simulink library "E78TestPack2"  (R2023b)
settings: Solver=VariableStepAuto  StartTime=0.0  StopTime=10.0  RelTol=1e-3
undefined symbols (not defined in the file or in its folder): battery_builder_rtmsupport, gcbh
libraries: E78TestPack2_lib x4
(part 2 of 2)

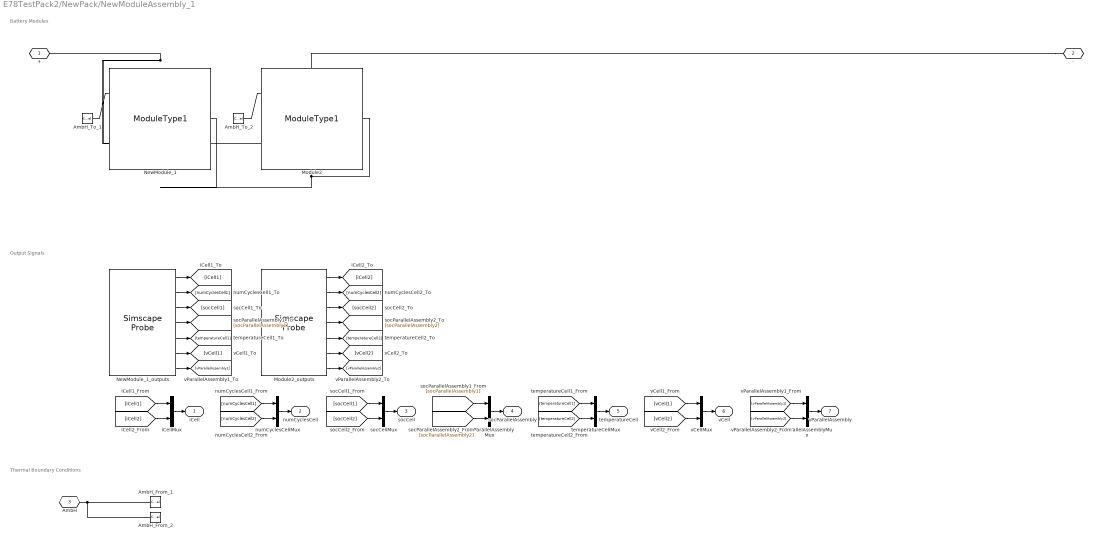
== system E78TestPack2/NewPack/NewModuleAssembly_1 ==
  note: Thermal Boundary Conditions
  note: Output Signals
  note: Battery Modules
  AmbH_From_1 : ConnectionLabel  Label=ambH_1
  AmbH_From_2 : ConnectionLabel  Label=ambH_2
  AmbH_To_1 : ConnectionLabel  Label=ambH_1
  AmbH_To_2 : ConnectionLabel  Label=ambH_2
  Module2 : E78TestPack2_lib/Modules/ModuleType1  SOC_vecCell=[0, .01, .02, .03, .04, .05, .06, .07, .08, .09, .1, .11, .12, .13, .14, .15, .16, .17, .18, .19, .2, .21, .22, .23, .24, .25, .26, .27, .28, .29, .3, .31, .32, .33, .34, .35, .36, .37, .38, .39, .4, .41, .42, .43, .44, .45, .46, .47, .48, .49, .5, .51, .52, .53, .54, .55, .56, .57, .58, .59, .6, .61, .62, .63, .64, .65, .66, .67, .68, .69, .7, .71, .72, .73, .74, .75, .76, .77, .78, .79, .8, .81, .82, .83, .84, .85, .86, .87, .88, .89, .9, .91, .92, .93, .94, .95, .96, .97, .98, .99, 1]  T_vecCell=[-10, 0, 10, 25, 35] degC  V0_matCell=[2.93217, 2.93217, 2.93217, 2.93217, 2.93217; 2.94263, 2.94263, 2.94263, 2.94263, 2.94263; 2.95309, 2.95309, 2.95309, 2.95309, 2.95309; 2.96355, 2.96355, 2.96355, 2.96355, 2.96355; 2.97401, 2.97401, 2.97401, 2.97401, 2.97401; 2.98447, 2.98447, 2.98447, 2.98447, 2.98447; 2.99493, 2.99493, 2.99493, 2.99493, 2.99493; 3.02455, 3.02455, 3.02455, 3.02455, 3.02455; 3.05382, 3.05382, 3.05382, 3.05382, 3.05382; 3.07377, 3.07377, 3.07377, 3.07377, 3.07377; 3.08453, 3.08453, 3.08453, 3.08453, 3.08453; 3.09529, 3.09529, 3.09529, 3.09529, 3.09529; 3.09916, 3.09916, 3.09916, 3.09916, 3.09916; 3.10271, 3.10271, 3.10271, 3.10271, 3.10271; 3.10625, 3.10625, 3.10625, 3.10625, 3.10625; 3.1098, 3.1098, 3.1098, 3.1098, 3.1098; 3.11335, 3.11335, 3.11335, 3.11335, 3.11335; 3.11689, 3.11689, 3.11689, 3.11689, 3.11689; 3.12044, 3.12044, 3.12044, 3.12044, 3.12044; 3.13089, 3.13089, 3.13089, 3.13089, 3.13089; 3.13795, 3.13795, 3.13795, 3.13795, 3.13795; 3.14459, 3.14459, 3.14459, 3.14459, 3.14459; 3.14961, 3.14961, 3.14961, 3.14961, 3.14961; 3.15451, 3.15451, 3.15451, 3.15451, 3.15451; 3.15932, 3.15932, 3.15932, 3.15932, 3.15932; 3.16324, 3.16324, 3.16324, 3.16324, 3.16324; 3.16716, 3.16716, 3.16716, 3.16716, 3.16716; 3.17063, 3.17063, 3.17063, 3.17063, 3.17063; 3.17297, 3.17297, 3.17297, 3.17297, 3.17297; 3.17544, 3.17544, 3.17544, 3.17544, 3.17544; 3.17798, 3.17798, 3.17798, 3.17798, 3.17798; 3.18052, 3.18052, 3.18052, 3.18052, 3.18052; 3.18295, 3.18295, 3.18295, 3.18295, 3.18295; 3.18533, 3.18533, 3.18533, 3.18533, 3.18533; 3.18771, 3.18771, 3.18771, 3.18771, 3.18771; 3.19009, 3.19009, 3.19009, 3.19009, 3.19009; 3.19215, 3.19215, 3.19215, 3.19215, 3.19215; 3.19403, 3.19403, 3.19403, 3.19403, 3.19403; 3.1959, 3.1959, 3.1959, 3.1959, 3.1959; 3.19777, 3.19777, 3.19777, 3.19777, 3.19777; 3.1998, 3.1998, 3.1998, 3.1998, 3.1998; 3.20198, 3.20198, 3.20198, 3.20198, 3.20198; 3.20371, 3.20371, 3.20371, 3.20371, 3.20371; 3.20501, 3.20501, 3.20501, 3.20501, 3.20501; 3.20619, 3.20619, 3.20619, 3.20619, 3.20619; 3.20738, 3.20738, 3.20738, 3.20738, 3.20738; 3.20856, 3.20856, 3.20856, 3.20856, 3.20856; 3.20974, 3.20974, 3.20974, 3.20974, 3.20974; 3.21092, 3.21092, 3.21092, 3.21092, 3.21092; 3.2121, 3.2121, 3.2121, 3.2121, 3.2121; 3.21329, 3.21329, 3.21329, 3.21329, 3.21329; 3.21447, 3.21447, 3.21447, 3.21447, 3.21447; 3.21565, 3.21565, 3.21565, 3.21565, 3.21565; 3.21672, 3.21672, 3.21672, 3.21672, 3.21672; 3.21787, 3.21787, 3.21787, 3.21787, 3.21787; 3.21904, 3.21904, 3.21904, 3.21904, 3.21904; 3.22021, 3.22021, 3.22021, 3.22021, 3.22021; 3.22139, 3.22139, 3.22139, 3.22139, 3.22139; 3.22256, 3.22256, 3.22256, 3.22256, 3.22256; 3.22374, 3.22374, 3.22374, 3.22374, 3.22374; 3.22492, 3.22492, 3.22492, 3.22492, 3.22492; 3.2261, 3.2261, 3.2261, 3.2261, 3.2261; 3.22728, 3.22728, 3.22728, 3.22728, 3.22728; 3.22847, 3.22847, 3.22847, 3.22847, 3.22847; 3.22965, 3.22965, 3.22965, 3.22965, 3.22965; 3.23083, 3.23083, 3.23083, 3.23083, 3.23083; 3.23201, 3.23201, 3.23201, 3.23201, 3.23201; 3.23319, 3.23319, 3.23319, 3.23319, 3.23319; 3.23437, 3.23437, 3.23437, 3.23437, 3.23437; 3.23552, 3.23552, 3.23552, 3.23552, 3.23552; 3.23652, 3.23652, 3.23652, 3.23652, 3.23652; 3.23778, 3.23778, 3.23778, 3.23778, 3.23778; 3.23909, 3.23909, 3.23909, 3.23909, 3.23909; 3.24045, 3.24045, 3.24045, 3.24045, 3.24045; 3.24217, 3.24217, 3.24217, 3.24217, 3.24217; 3.2439, 3.2439, 3.2439, 3.2439, 3.2439; 3.24563, 3.24563, 3.24563, 3.24563, 3.24563; 3.24736, 3.24736, 3.24736, 3.24736, 3.24736; 3.24909, 3.24909, 3.24909, 3.24909, 3.24909; 3.25082, 3.25082, 3.25082, 3.25082, 3.25082; 3.25255, 3.25255, 3.25255, 3.25255, 3.25255; 3.25428, 3.25428, 3.25428, 3.25428, 3.25428; 3.256, 3.256, 3.256, 3.256, 3.256; 3.25774, 3.25774, 3.25774, 3.25774, 3.25774; 3.25951, 3.25951, 3.25951, 3.25951, 3.25951; 3.26116, 3.26116, 3.26116, 3.26116, 3.26116; 3.26238, 3.26238, 3.26238, 3.26238, 3.26238; 3.26307, 3.26307, 3.26307, 3.26307, 3.26307; 3.26352, 3.26352, 3.26352, 3.26352, 3.26352; 3.26396, 3.26396, 3.26396, ...(+502 chars)] V  V_rangeCell=[1.8, Inf] V  R0_matCell=[.07996, .07435, .07218, .00349, .04758; .07879, .07234, .06844, .0033, .01888; .07763, .07033, .0647, .00311, .01407; .07646, .06833, .06096, .00292, .00948; .07529, .06632, .05722, .00272, .0049; .07413, .06432, .05347, .00253, .00119; .07296, .06231, .04973, .00235, .00022; .07278, .06129, .04698, .00233, .00024; .07258, .06024, .0446, .00235, .00024; .0719, .05873, .04247, .00232, .00024; .07075, .05673, .03988, .00223, .00024; .0696, .05474, .03743, .00214, .00024; .06809, .0524, .03472, .00205, .00024; .06657, .05004, .032, .00196, .00024; .06505, .04768, .02927, .00187, .00024; .06353, .04532, .02655, .00181, .00024; .06201, .04298, .02426, .00175, .00024; .06049, .04073, .02215, .00169, .00024; .05897, .03848, .02004, .00164, .00024; .0578, .03658, .01828, .00167, .0006; .05646, .03451, .01635, .00168, .00078; .0551, .03261, .01479, .00168, .00094; .05366, .03068, .01317, .00168, .00101; .0522, .02875, .01154, .00168, .00108; .05075, .02681, .01054, .00167, .00114; .04925, .02502, .01001, .00167, .00116; .04759, .02356, .00948, .00167, .00118; .04591, .02208, .00893, .00167, .00118; .04416, .02054, .00832, .00166, .00112; .04243, .01901, .00772, .00165, .00111; .0407, .01812, .00742, .00164, .00113; .03899, .01727, .0072, .00164, .00115; .03731, .01641, .00697, .00163, .00116; .03563, .01555, .00675, .00163, .00117; .03395, .01474, .00652, .00162, .00119; .03227, .01421, .0063, .00162, .0012; .03067, .01366, .00605, .00161, .00119; .02945, .0131, .00583, .0016, .00118; .02823, .01254, .0058, .00159, .00117; .02701, .01213, .00577, .00159, .00115; .02586, .01192, .00574, .00158, .00115; .02512, .01173, .00573, .00158, .00115; .02436, .01151, .00569, .00158, .00113; .02358, .01127, .00563, .00157, .00109; .02279, .01107, .00557, .00156, .00111; .022, .01096, .0055, .00156, .00112; .02121, .01085, .00544, .00155, .00114; .02046, .01074, .00537, .00154, .00115; .0201, .01063, .00534, .00154, .00117; .01974, .01052, .00531, .00153, .00118; .01938, .01042, .00528, .00153, .00119; .01902, .01031, .00526, .00152, .00121; .01865, .0102, .00523, .00151, .00122; .01829, .01009, .00519, .00151, .00123; .01792, .00998, .00516, .0015, .00124; .01756, .00987, .00513, .0015, .00126; .01735, .00976, .0051, .0015, .00127; .01723, .00967, .00507, .00149, .00128; .01712, .00965, .00504, .00149, .0013; .017, .00963, .00501, .00149, .00131; .01688, .00961, .00498, .00148, .00133; .01676, .00959, .00496, .00148, .00134; .01665, .00957, .00493, .00148, .00135; .01653, .00955, .0049, .00147, .00137; .01641, .00953, .00488, .00147, .00138; .01629, .00951, .00485, .00147, .0014; .01618, .00949, .00482, .00147, .00141; .01606, .00947, .00479, .00146, .00142; .01594, .00945, .00477, .00146, .00143; .01589, .00942, .00474, .00146, .00141; .01586, .00937, .0047, .00145, .00139; .01584, .00934, .00468, .00146, .00139; .01583, .0093, .00466, .00146, .00138; .01581, .00927, .00464, .00147, .00138; .01582, .00926, .00464, .00147, .0014; .01583, .00925, .00464, .00148, .00141; .01583, .00924, .00465, .00149, .00143; .01584, .00923, .00465, .0015, .00145; .01584, .00921, .00465, .0015, .00146; .01585, .00923, .00465, .00151, .00148; .01585, .00925, .00465, .00152, .0015; .01586, .00926, .00465, .00153, .00152; .01587, .00928, .00465, .00153, .00153; .01587, .0093, .00464, .00154, .00155; .01588, .00932, .00463, .00155, .00157; .01589, .00933, .00462, .00155, .00158; .01587, .00933, .00459, .00156, .00157; .01582, .00929, .00453, .00155, .00154; .01576, .00924, .00446, .00154, .00146; .0157, .00919, .00438, .00153, .00132; .01564, .00915, .00431, .00152, .00118; .01558, .0091, .00424, .00151, .00103; .01552, .00905, .00416, .0015, .00089; .01539, .00891, .0041, .00148, .00076; .01518, .00871, .00401, .00144, .00061; .01502, .00857, .00398, .0014, .00051; .01487, .00844, .00396, .00137, .00041; .01501, .0086, .00385, .00136, .00062; .01436, .00795, .00371, .00131, .00087; .01329, .00785, .00411, .00127, .00126; .01299, .00622, .00111, .00104, .00185] Ohm  AHCell=19.487 A*hr  extrapolation_optionCell=simscape.enum.extrapolation.nearest  thermal_massCell=446.4 J/K  AmbientResistance=25 K/W  InterParallelAssemblyThermalResistance=1 K/W  InterParallelAssemblyRadiationArea=1e-3 m^2  InterParallelAssemblyRadiationCoefficient=1e-6 W/(K^4*m^2)  P=1  S=12  NumInterParallelAssemblyThermalConnections=11  InterParallelAssemblyConnectionsMapping=[1, 2, 3, 4, 5, 6, 7, 8, 9, 10, 11; 2, 3, 4, 5, 6, 7, 8, 9, 10, 11, 12]  InterParallelAssemblyCellConnectionsMapping=[1, 1, 1, 1, 1, 1, 1, 1, 1, 1, 1; 1, 1, 1, 1, 1, 1, 1, 1, 1, 1, 1]  iCell_specify=off  iCell_priority=None  iCell=repmat(0, 12, 1) A  iCell_nominal_specify=off  iCell_nominal_unit=A  iCell_nominal_value=1  vCell_specify=off  vCell_priority=None  vCell=repmat(0, 12, 1) V  vCell_nominal_specify=off  vCell_nominal_unit=V  vCell_nominal_value=1  socCell_specify=off  socCell_priority=High  socCell=repmat(1, 12, 1)  socCell_nominal_specify=off  socCell_nominal_unit=1  socCell_nominal_value=1  numCyclesCell_specify=off  numCyclesCell_priority=High  numCyclesCell=repmat(0, 12, 1)  numCyclesCell_nominal_specify=off  numCyclesCell_nominal_unit=1  numCyclesCell_nominal_value=1  temperatureCell_specify=off  temperatureCell_priority=High  temperatureCell=repmat(298.15, 12, 1) K  temperatureCell_nominal_specify=off  temperatureCell_nominal_unit=K  temperatureCell_nominal_value=1  vParallelAssembly_specify=off  vParallelAssembly_priority=None  vParallelAssembly=repmat(0, 12, 1) V  vParallelAssembly_nominal_specify=off  vParallelAssembly_nominal_unit=V  vParallelAssembly_nominal_value=1  socParallelAssembly_specify=off  socParallelAssembly_priority=None  socParallelAssembly=repmat(1, 12, 1)  socParallelAssembly_nominal_specify=off  socParallelAssembly_nominal_unit=1  socParallelAssembly_nominal_value=1
      settings: InternalSimscapePortConfiguration="{\"Bottom\":[{\"id\":\"n\",\"label\":\"-\",\"type\":\"foundation.electrical.electrical\"}],\"Left\":[{\"id\":\"AmbH\",\"label\":\"AmbH\",\"type\":\"foundation.thermal.thermal\"}],\"Right\":[],\"Top\":[{\"id\":\"p\",\"label\":\"+\",\"type\":\"foundation.electrical.electrical\"}]}"
  Module2_outputs : SimscapeProbe  BoundBlock=65  Variables={iCell, numCyclesCell, socCell, socParallelAssembly, temperatureCell, vCell, vParallelAssembly}
  NewModule_1 : E78TestPack2_lib/Modules/ModuleType1  SOC_vecCell=[0, .01, .02, .03, .04, .05, .06, .07, .08, .09, .1, .11, .12, .13, .14, .15, .16, .17, .18, .19, .2, .21, .22, .23, .24, .25, .26, .27, .28, .29, .3, .31, .32, .33, .34, .35, .36, .37, .38, .39, .4, .41, .42, .43, .44, .45, .46, .47, .48, .49, .5, .51, .52, .53, .54, .55, .56, .57, .58, .59, .6, .61, .62, .63, .64, .65, .66, .67, .68, .69, .7, .71, .72, .73, .74, .75, .76, .77, .78, .79, .8, .81, .82, .83, .84, .85, .86, .87, .88, .89, .9, .91, .92, .93, .94, .95, .96, .97, .98, .99, 1]  T_vecCell=[-10, 0, 10, 25, 35] degC  V0_matCell=[2.93217, 2.93217, 2.93217, 2.93217, 2.93217; 2.94263, 2.94263, 2.94263, 2.94263, 2.94263; 2.95309, 2.95309, 2.95309, 2.95309, 2.95309; 2.96355, 2.96355, 2.96355, 2.96355, 2.96355; 2.97401, 2.97401, 2.97401, 2.97401, 2.97401; 2.98447, 2.98447, 2.98447, 2.98447, 2.98447; 2.99493, 2.99493, 2.99493, 2.99493, 2.99493; 3.02455, 3.02455, 3.02455, 3.02455, 3.02455; 3.05382, 3.05382, 3.05382, 3.05382, 3.05382; 3.07377, 3.07377, 3.07377, 3.07377, 3.07377; 3.08453, 3.08453, 3.08453, 3.08453, 3.08453; 3.09529, 3.09529, 3.09529, 3.09529, 3.09529; 3.09916, 3.09916, 3.09916, 3.09916, 3.09916; 3.10271, 3.10271, 3.10271, 3.10271, 3.10271; 3.10625, 3.10625, 3.10625, 3.10625, 3.10625; 3.1098, 3.1098, 3.1098, 3.1098, 3.1098; 3.11335, 3.11335, 3.11335, 3.11335, 3.11335; 3.11689, 3.11689, 3.11689, 3.11689, 3.11689; 3.12044, 3.12044, 3.12044, 3.12044, 3.12044; 3.13089, 3.13089, 3.13089, 3.13089, 3.13089; 3.13795, 3.13795, 3.13795, 3.13795, 3.13795; 3.14459, 3.14459, 3.14459, 3.14459, 3.14459; 3.14961, 3.14961, 3.14961, 3.14961, 3.14961; 3.15451, 3.15451, 3.15451, 3.15451, 3.15451; 3.15932, 3.15932, 3.15932, 3.15932, 3.15932; 3.16324, 3.16324, 3.16324, 3.16324, 3.16324; 3.16716, 3.16716, 3.16716, 3.16716, 3.16716; 3.17063, 3.17063, 3.17063, 3.17063, 3.17063; 3.17297, 3.17297, 3.17297, 3.17297, 3.17297; 3.17544, 3.17544, 3.17544, 3.17544, 3.17544; 3.17798, 3.17798, 3.17798, 3.17798, 3.17798; 3.18052, 3.18052, 3.18052, 3.18052, 3.18052; 3.18295, 3.18295, 3.18295, 3.18295, 3.18295; 3.18533, 3.18533, 3.18533, 3.18533, 3.18533; 3.18771, 3.18771, 3.18771, 3.18771, 3.18771; 3.19009, 3.19009, 3.19009, 3.19009, 3.19009; 3.19215, 3.19215, 3.19215, 3.19215, 3.19215; 3.19403, 3.19403, 3.19403, 3.19403, 3.19403; 3.1959, 3.1959, 3.1959, 3.1959, 3.1959; 3.19777, 3.19777, 3.19777, 3.19777, 3.19777; 3.1998, 3.1998, 3.1998, 3.1998, 3.1998; 3.20198, 3.20198, 3.20198, 3.20198, 3.20198; 3.20371, 3.20371, 3.20371, 3.20371, 3.20371; 3.20501, 3.20501, 3.20501, 3.20501, 3.20501; 3.20619, 3.20619, 3.20619, 3.20619, 3.20619; 3.20738, 3.20738, 3.20738, 3.20738, 3.20738; 3.20856, 3.20856, 3.20856, 3.20856, 3.20856; 3.20974, 3.20974, 3.20974, 3.20974, 3.20974; 3.21092, 3.21092, 3.21092, 3.21092, 3.21092; 3.2121, 3.2121, 3.2121, 3.2121, 3.2121; 3.21329, 3.21329, 3.21329, 3.21329, 3.21329; 3.21447, 3.21447, 3.21447, 3.21447, 3.21447; 3.21565, 3.21565, 3.21565, 3.21565, 3.21565; 3.21672, 3.21672, 3.21672, 3.21672, 3.21672; 3.21787, 3.21787, 3.21787, 3.21787, 3.21787; 3.21904, 3.21904, 3.21904, 3.21904, 3.21904; 3.22021, 3.22021, 3.22021, 3.22021, 3.22021; 3.22139, 3.22139, 3.22139, 3.22139, 3.22139; 3.22256, 3.22256, 3.22256, 3.22256, 3.22256; 3.22374, 3.22374, 3.22374, 3.22374, 3.22374; 3.22492, 3.22492, 3.22492, 3.22492, 3.22492; 3.2261, 3.2261, 3.2261, 3.2261, 3.2261; 3.22728, 3.22728, 3.22728, 3.22728, 3.22728; 3.22847, 3.22847, 3.22847, 3.22847, 3.22847; 3.22965, 3.22965, 3.22965, 3.22965, 3.22965; 3.23083, 3.23083, 3.23083, 3.23083, 3.23083; 3.23201, 3.23201, 3.23201, 3.23201, 3.23201; 3.23319, 3.23319, 3.23319, 3.23319, 3.23319; 3.23437, 3.23437, 3.23437, 3.23437, 3.23437; 3.23552, 3.23552, 3.23552, 3.23552, 3.23552; 3.23652, 3.23652, 3.23652, 3.23652, 3.23652; 3.23778, 3.23778, 3.23778, 3.23778, 3.23778; 3.23909, 3.23909, 3.23909, 3.23909, 3.23909; 3.24045, 3.24045, 3.24045, 3.24045, 3.24045; 3.24217, 3.24217, 3.24217, 3.24217, 3.24217; 3.2439, 3.2439, 3.2439, 3.2439, 3.2439; 3.24563, 3.24563, 3.24563, 3.24563, 3.24563; 3.24736, 3.24736, 3.24736, 3.24736, 3.24736; 3.24909, 3.24909, 3.24909, 3.24909, 3.24909; 3.25082, 3.25082, 3.25082, 3.25082, 3.25082; 3.25255, 3.25255, 3.25255, 3.25255, 3.25255; 3.25428, 3.25428, 3.25428, 3.25428, 3.25428; 3.256, 3.256, 3.256, 3.256, 3.256; 3.25774, 3.25774, 3.25774, 3.25774, 3.25774; 3.25951, 3.25951, 3.25951, 3.25951, 3.25951; 3.26116, 3.26116, 3.26116, 3.26116, 3.26116; 3.26238, 3.26238, 3.26238, 3.26238, 3.26238; 3.26307, 3.26307, 3.26307, 3.26307, 3.26307; 3.26352, 3.26352, 3.26352, 3.26352, 3.26352; 3.26396, 3.26396, 3.26396, ...(+502 chars)] V  V_rangeCell=[1.8, Inf] V  R0_matCell=[.07996, .07435, .07218, .00349, .04758; .07879, .07234, .06844, .0033, .01888; .07763, .07033, .0647, .00311, .01407; .07646, .06833, .06096, .00292, .00948; .07529, .06632, .05722, .00272, .0049; .07413, .06432, .05347, .00253, .00119; .07296, .06231, .04973, .00235, .00022; .07278, .06129, .04698, .00233, .00024; .07258, .06024, .0446, .00235, .00024; .0719, .05873, .04247, .00232, .00024; .07075, .05673, .03988, .00223, .00024; .0696, .05474, .03743, .00214, .00024; .06809, .0524, .03472, .00205, .00024; .06657, .05004, .032, .00196, .00024; .06505, .04768, .02927, .00187, .00024; .06353, .04532, .02655, .00181, .00024; .06201, .04298, .02426, .00175, .00024; .06049, .04073, .02215, .00169, .00024; .05897, .03848, .02004, .00164, .00024; .0578, .03658, .01828, .00167, .0006; .05646, .03451, .01635, .00168, .00078; .0551, .03261, .01479, .00168, .00094; .05366, .03068, .01317, .00168, .00101; .0522, .02875, .01154, .00168, .00108; .05075, .02681, .01054, .00167, .00114; .04925, .02502, .01001, .00167, .00116; .04759, .02356, .00948, .00167, .00118; .04591, .02208, .00893, .00167, .00118; .04416, .02054, .00832, .00166, .00112; .04243, .01901, .00772, .00165, .00111; .0407, .01812, .00742, .00164, .00113; .03899, .01727, .0072, .00164, .00115; .03731, .01641, .00697, .00163, .00116; .03563, .01555, .00675, .00163, .00117; .03395, .01474, .00652, .00162, .00119; .03227, .01421, .0063, .00162, .0012; .03067, .01366, .00605, .00161, .00119; .02945, .0131, .00583, .0016, .00118; .02823, .01254, .0058, .00159, .00117; .02701, .01213, .00577, .00159, .00115; .02586, .01192, .00574, .00158, .00115; .02512, .01173, .00573, .00158, .00115; .02436, .01151, .00569, .00158, .00113; .02358, .01127, .00563, .00157, .00109; .02279, .01107, .00557, .00156, .00111; .022, .01096, .0055, .00156, .00112; .02121, .01085, .00544, .00155, .00114; .02046, .01074, .00537, .00154, .00115; .0201, .01063, .00534, .00154, .00117; .01974, .01052, .00531, .00153, .00118; .01938, .01042, .00528, .00153, .00119; .01902, .01031, .00526, .00152, .00121; .01865, .0102, .00523, .00151, .00122; .01829, .01009, .00519, .00151, .00123; .01792, .00998, .00516, .0015, .00124; .01756, .00987, .00513, .0015, .00126; .01735, .00976, .0051, .0015, .00127; .01723, .00967, .00507, .00149, .00128; .01712, .00965, .00504, .00149, .0013; .017, .00963, .00501, .00149, .00131; .01688, .00961, .00498, .00148, .00133; .01676, .00959, .00496, .00148, .00134; .01665, .00957, .00493, .00148, .00135; .01653, .00955, .0049, .00147, .00137; .01641, .00953, .00488, .00147, .00138; .01629, .00951, .00485, .00147, .0014; .01618, .00949, .00482, .00147, .00141; .01606, .00947, .00479, .00146, .00142; .01594, .00945, .00477, .00146, .00143; .01589, .00942, .00474, .00146, .00141; .01586, .00937, .0047, .00145, .00139; .01584, .00934, .00468, .00146, .00139; .01583, .0093, .00466, .00146, .00138; .01581, .00927, .00464, .00147, .00138; .01582, .00926, .00464, .00147, .0014; .01583, .00925, .00464, .00148, .00141; .01583, .00924, .00465, .00149, .00143; .01584, .00923, .00465, .0015, .00145; .01584, .00921, .00465, .0015, .00146; .01585, .00923, .00465, .00151, .00148; .01585, .00925, .00465, .00152, .0015; .01586, .00926, .00465, .00153, .00152; .01587, .00928, .00465, .00153, .00153; .01587, .0093, .00464, .00154, .00155; .01588, .00932, .00463, .00155, .00157; .01589, .00933, .00462, .00155, .00158; .01587, .00933, .00459, .00156, .00157; .01582, .00929, .00453, .00155, .00154; .01576, .00924, .00446, .00154, .00146; .0157, .00919, .00438, .00153, .00132; .01564, .00915, .00431, .00152, .00118; .01558, .0091, .00424, .00151, .00103; .01552, .00905, .00416, .0015, .00089; .01539, .00891, .0041, .00148, .00076; .01518, .00871, .00401, .00144, .00061; .01502, .00857, .00398, .0014, .00051; .01487, .00844, .00396, .00137, .00041; .01501, .0086, .00385, .00136, .00062; .01436, .00795, .00371, .00131, .00087; .01329, .00785, .00411, .00127, .00126; .01299, .00622, .00111, .00104, .00185] Ohm  AHCell=19.487 A*hr  extrapolation_optionCell=simscape.enum.extrapolation.nearest  thermal_massCell=446.4 J/K  AmbientResistance=25 K/W  InterParallelAssemblyThermalResistance=1 K/W  InterParallelAssemblyRadiationArea=1e-3 m^2  InterParallelAssemblyRadiationCoefficient=1e-6 W/(K^4*m^2)  P=1  S=12  NumInterParallelAssemblyThermalConnections=11  InterParallelAssemblyConnectionsMapping=[1, 2, 3, 4, 5, 6, 7, 8, 9, 10, 11; 2, 3, 4, 5, 6, 7, 8, 9, 10, 11, 12]  InterParallelAssemblyCellConnectionsMapping=[1, 1, 1, 1, 1, 1, 1, 1, 1, 1, 1; 1, 1, 1, 1, 1, 1, 1, 1, 1, 1, 1]  iCell_specify=off  iCell_priority=None  iCell=repmat(0, 12, 1) A  iCell_nominal_specify=off  iCell_nominal_unit=A  iCell_nominal_value=1  vCell_specify=off  vCell_priority=None  vCell=repmat(0, 12, 1) V  vCell_nominal_specify=off  vCell_nominal_unit=V  vCell_nominal_value=1  socCell_specify=off  socCell_priority=High  socCell=repmat(1, 12, 1)  socCell_nominal_specify=off  socCell_nominal_unit=1  socCell_nominal_value=1  numCyclesCell_specify=off  numCyclesCell_priority=High  numCyclesCell=repmat(0, 12, 1)  numCyclesCell_nominal_specify=off  numCyclesCell_nominal_unit=1  numCyclesCell_nominal_value=1  temperatureCell_specify=off  temperatureCell_priority=High  temperatureCell=repmat(298.15, 12, 1) K  temperatureCell_nominal_specify=off  temperatureCell_nominal_unit=K  temperatureCell_nominal_value=1  vParallelAssembly_specify=off  vParallelAssembly_priority=None  vParallelAssembly=repmat(0, 12, 1) V  vParallelAssembly_nominal_specify=off  vParallelAssembly_nominal_unit=V  vParallelAssembly_nominal_value=1  socParallelAssembly_specify=off  socParallelAssembly_priority=None  socParallelAssembly=repmat(1, 12, 1)  socParallelAssembly_nominal_specify=off  socParallelAssembly_nominal_unit=1  socParallelAssembly_nominal_value=1
      settings: InternalSimscapePortConfiguration="{\"Bottom\":[{\"id\":\"n\",\"label\":\"-\",\"type\":\"foundation.electrical.electrical\"}],\"Left\":[{\"id\":\"AmbH\",\"label\":\"AmbH\",\"type\":\"foundation.thermal.thermal\"}],\"Right\":[],\"Top\":[{\"id\":\"p\",\"label\":\"+\",\"type\":\"foundation.electrical.electrical\"}]}"
  NewModule_1_outputs : SimscapeProbe  BoundBlock=67  Variables={iCell, numCyclesCell, socCell, socParallelAssembly, temperatureCell, vCell, vParallelAssembly}
  iCellMux : Mux  Inputs=2
  numCyclesCellMux : Mux  Inputs=2
  socCellMux : Mux  Inputs=2
  socParallelAssemblyMux : Mux  Inputs=2
  temperatureCellMux : Mux  Inputs=2
  vCellMux : Mux  Inputs=2
  vParallelAssemblyMux : Mux  Inputs=2
  + : PMIOPort  Side=Left
  - : PMIOPort  Port=2  Side=Right
  AmbH : PMIOPort  Port=3  Side=Right  ConnectionType=Connection: foundation.thermal.thermal
  iCell : Outport
  numCyclesCell : Outport  Port=2
  socCell : Outport  Port=3
  socParallelAssembly : Outport  Port=4
  temperatureCell : Outport  Port=5
  vCell : Outport  Port=6
  vParallelAssembly : Outport  Port=7
  wires:
  [vParallelAssembly2] -> vParallelAssemblyMux/2
  Module2_outputs/7 -> [vParallelAssembly2]
  [vCell2] -> vCellMux/2
  Module2_outputs/6 -> [vCell2]
  [temperatureCell2] -> temperatureCellMux/2
  Module2_outputs/5 -> [temperatureCell2]
  [socParallelAssembly2] -> socParallelAssemblyMux/2
  Module2_outputs/4 -> [socParallelAssembly2]
  [socCell2] -> socCellMux/2
  Module2_outputs/3 -> [socCell2]
  [numCyclesCell2] -> numCyclesCellMux/2
  Module2_outputs/2 -> [numCyclesCell2]
  [iCell2] -> iCellMux/2
  Module2_outputs/1 -> [iCell2]
  [vParallelAssembly1] -> vParallelAssemblyMux/1
  vParallelAssemblyMux/1 -> vParallelAssembly/1
  NewModule_1_outputs/7 -> [vParallelAssembly1]
  [vCell1] -> vCellMux/1
  vCellMux/1 -> vCell/1
  NewModule_1_outputs/6 -> [vCell1]
  [temperatureCell1] -> temperatureCellMux/1
  temperatureCellMux/1 -> temperatureCell/1
  NewModule_1_outputs/5 -> [temperatureCell1]
  [socParallelAssembly1] -> socParallelAssemblyMux/1
  socParallelAssemblyMux/1 -> socParallelAssembly/1
  NewModule_1_outputs/4 -> [socParallelAssembly1]
  [socCell1] -> socCellMux/1
  socCellMux/1 -> socCell/1
  NewModule_1_outputs/3 -> [socCell1]
  [numCyclesCell1] -> numCyclesCellMux/1
  numCyclesCellMux/1 -> numCyclesCell/1
  NewModule_1_outputs/2 -> [numCyclesCell1]
  [iCell1] -> iCellMux/1
  iCellMux/1 -> iCell/1
  NewModule_1_outputs/1 -> [iCell1]
  connections:
  AmbH_To_2/LConn1 -- Module2/LConn1
  AmbH_From_2/LConn1 -- AmbH_From_1/LConn1 -- AmbH/RConn1
  AmbH_To_1/LConn1 -- NewModule_1/LConn1
  -/RConn1 -- Module2/RConn1 -- NewModule_1/RConn1
  +/RConn1 -- Module2/LConn2 -- NewModule_1/LConn2
